simulink model "mass_spring"  (Simulink 8.0)
settings: Solver=ode45  StartTime=0.0  StopTime=10.0  RelTol=1e-3
settings Model: Creator=Vaio  LastModifiedBy=Tran Minh Luan
settings DataIOCC: SignalLoggingSaveFormat=ModelDataLogs
settings DebuggingCC: FcnCallInpInsideContextMsg=EnableAllAsWarning

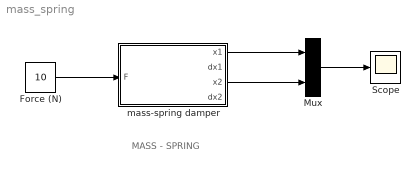
== system mass_spring ==
  note: MASS - SPRING
  Force (N) : Constant  Value=10
  Mux : Mux  Inputs=2
  Scope : Scope
  mass-spring damper : Subsystem
  wires:
  Force (N)/1 -> mass-spring damper/1(F)
  mass-spring damper/1(x1) -> Mux/1
  mass-spring damper/3(x2) -> Mux/2
  Mux/1 -> Scope/1

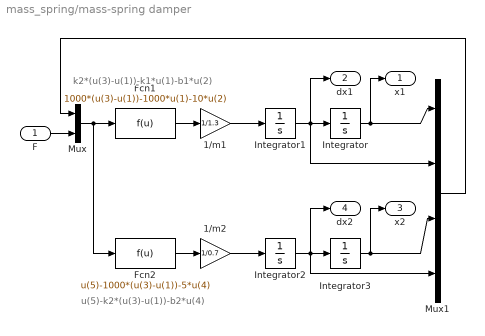
== system mass_spring/mass-spring damper ==
  note: u(5)-k2*(u(3)-u(1))-b2*u(4)
  note: k2*(u(3)-u(1))-k1*u(1)-b1*u(2)
  F : Inport
  1/m1 : Gain  Gain=1/1.3
  1/m2 : Gain  Gain=1/0.7
  "Fcn1 " : Fcn  Expr=1000*(u(3)-u(1))-1000*u(1)-10*u(2)
  "Fcn2 " : Fcn  Expr=u(5)-1000*(u(3)-u(1))-5*u(4)
  Integrator{,1..3} (4 alike) : Integrator
  Mux : Mux  Inputs=2
  Mux1 : Mux
  x1 : Outport
  dx1 : Outport  Port=2
  x2 : Outport  Port=3
  dx2 : Outport  Port=4
  wires:
  F/1 -> Mux/2
  1/m1/1 -> Integrator1/1
  Integrator1/1 -> Integrator/1, dx1/1, Mux1/2
  Integrator/1 -> Mux1/1, x1/1
  Integrator3/1 -> Mux1/3, x2/1
  Integrator2/1 -> Integrator3/1, dx2/1, Mux1/4
  1/m2/1 -> Integrator2/1
  Mux1/1 -> Mux/1
  Mux/1 -> "Fcn2 "/1, "Fcn1 "/1
  "Fcn1 "/1 -> 1/m1/1
  "Fcn2 "/1 -> 1/m2/1
